simulink model "EV_model"  (R2020a)
settings: Solver=VariableStepAuto  StartTime=0  StopTime=length_DriveCycle* n_repeat  FixedStep=1  RelTol=1e-3
model workspace (MAT data in the model file):
  Af = 4
  Cd = 0.3
  DrCycles.C505 = [0 1 2 3 4 5 6 7 8 9 10 11 ... (1012 elements, 506x2)]
  DrCycles.FTP = [0 1 2 3 4 5 6 7 8 9 10 11 ... (4956 elements, 2478x2)]
  DrCycles.UDDS = [0 1 2 3 4 5 6 7 8 9 10 11 ... (2746 elements, 1373x2)]
  DrCycles.HWFET = [0 1 2 3 4 5 6 7 8 9 10 11 ... (1532 elements, 766x2)]
  DrCycles.US06 = [0 1 2 3 4 5 6 7 8 9 10 11 ... (1194 elements, 597x2)]
  DrCycles.US06City = [0 1 2 3 4 5 6 7 8 9 10 11 ... (466 elements, 233x2)]
  DrCycles.US06Hwy = [0 1 2 3 4 5 6 7 8 9 10 11 ... (742 elements, 371x2)]
  I = 1
  Kbr = 5000
  P = 20
  TimeHWFET = 765
  TimeUDDS = 1372
  TimeUS06 = 596
  axle_b = 10
  axle_k = 5000
  bevAxle_wc = 400
  bevNp = 2
  bevNs = 30
  diffRatio = 3.4
  diffRatio1 = 3.4
  motorMaxTorqueNm = [500 500 500 500 500 500 416.666666667 357.142857143 312.5 277.777777778 250 227.272727273 208.333333333 192.307692308 178.571428571 166.666666667]
  motorSpeedRadPs = [0 40 80 120 160 200 240 280 320 360 400 440 480 520 560 600]
  vehicleMass = 1500
  wheelRadius = 0.35
values from neighbouring files (symbols this model uses):
  b = 4.48/2    (= 2.24)    [NissanLeaf_input_data.m]    (also in TeslaS_input_data.m = 2.5)
  Ct = Cp_cell*rho_cell*cell_volume    (= 2759947.2)    [NissanLeaf_input_data.m]    (also in TeslaS_input_data.m = 37.7660192772)
  driving_range = 363    [NissanLeaf_input_data.m]    (also in TeslaS_input_data.m = 600)
  m = 1789    [NissanLeaf_input_data.m]    (also in TeslaS_input_data.m = 2250)
  motorMaxTorqueNm_my = [340 340 340 340 340 340 300 260  230  210 190   175 160 150 140 130 125 120]    [NissanLeaf_input_data.m]    (also in TeslaS_input_data.m = [660 660 660 660 660 660 550 475 400 325 275 225 200 175 150)
  motorSpeedRadPs_my = [1000 1500 2000 2500 3000 3250 3500 4000 4500 5000 5500 6000 6500  7000 7500 8000 8500 9000]*transRatio*2*pi/60    [NissanLeaf_input_data.m]    (also in TeslaS_input_data.m = [0 10 20 30 40 50 60 70 80 90 100 110 120 130 140 150]*0.447)
  regen_eff = 0.7    [NissanLeaf_input_data.m]    (also in TeslaS_input_data.m)
  Rt = 0.01    [NissanLeaf_input_data.m]    (also in TeslaS_input_data.m = 0.316348525327)
  T = 20    [NissanLeaf_input_data.m]    (also in TeslaS_input_data.m = 25; battery_parametrization.m)
  transRatio = 8.19    [NissanLeaf_input_data.m]    (also in TeslaS_input_data.m = 9.3)
undefined symbols (not defined in the file or in its folder): Driver, Wheels_Driver_VehDyn_Lib
libraries: autolibshared x3, simulink x2, autolibdatasheetbattery x1, autolibmappedmotor x1, autolibsharedcoupling x1, autolibshareddiff x1
(part 1 of 3)
settings Model: PauseTimes=2  Creator=ogden.michael  LastModifiedBy=marcoragone-macbookpro
settings SolverCC: AlgebraicLoopSolver=LineSearch
settings DataIOCC: ReturnWorkspaceOutputs=off
settings DebuggingCC: AlgebraicLoopMsg=none  ArithmeticOperatorsInVariantConditions=warning
settings SFSimCC: SimUseLocalCustomCode=off  CustomCodeUndefinedFunction=UseInterfaceOnly
settings RTWCC: RTWUseLocalCustomCode=off
settings CodeAppCC: StateflowObjectComments=on
settings SimscapeCC: SimscapeNormalizeSystem=off

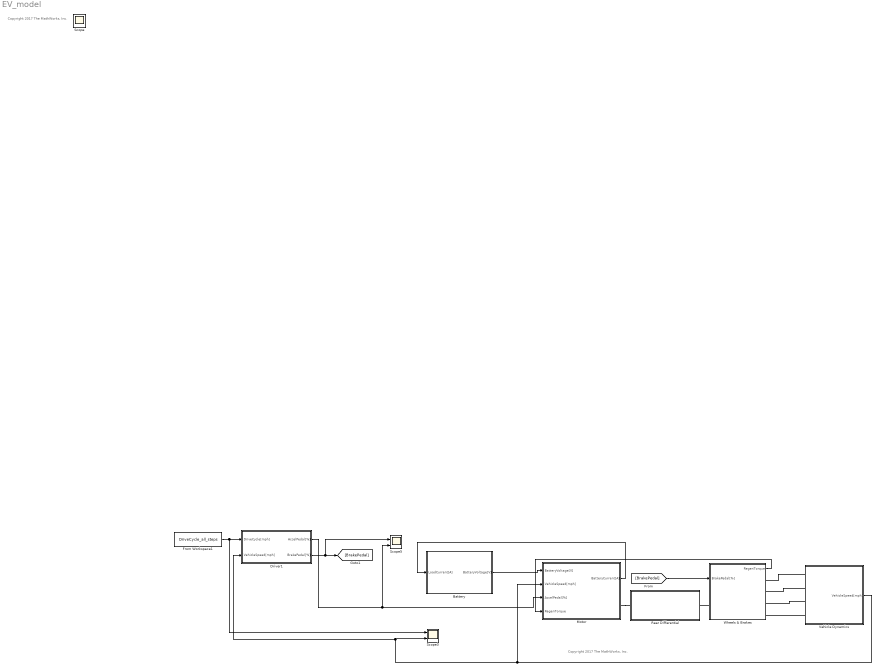
== system EV_model ==
  note: Copyright 2017 The MathWorks, Inc.
  note: Copyright 2017 The MathWorks, Inc.
  Battery : Subsystem
  Driver1 : Subsystem  AncestorBlock=Wheels_Driver_VehDyn_Lib/Driver
  From Workspace1 : FromWorkspace  VariableName=DriveCycle_all_steps
  Motor : Subsystem
  Rear Differential : Subsystem
  Scope3 : Scope  NumInputPorts=2
  Scope5 : Scope  NumInputPorts=2
  Vehicle Dynamics : Subsystem  AncestorBlock=Wheels_Driver_VehDyn_Lib/Vehicle Dynamics
  Wheels & Brakes : Subsystem  AncestorBlock=Wheels_Driver_VehDyn_Lib/Wheels & Brakes
  Scope : Scope
  wires:
  [BrakePedal] -> Wheels & Brakes/1(BrakePedal[%])
  Battery/1(BatteryVoltage[V]) -> Motor/1(BatteryVoltage[V])
  Vehicle Dynamics/1(VehicleSpeed[mph]) -> Scope3/2, Driver1/2(VehicleSpeed[mph]), Motor/2(VehicleSpeed[mph])
  Driver1/1(AccelPedal[%]) -> Scope5/2, Motor/3(AccelPedal[%])
  From Workspace1/1 -> Scope3/1, Driver1/1(" DriveCycle[mph]")
  Driver1/2(BrakePedal[%]) -> Scope5/1, [BrakePedal]
  Motor/1(BatteryCurrent[A]) -> Battery/1(LoadCurrent[A])
  Wheels & Brakes/1(RegenTorque) -> Motor/4(RegenTorque)
  connections:
  Motor/RConn1 -- Rear Differential/LConn1
  Wheels & Brakes/LConn1 -- Rear Differential/RConn1
  Vehicle Dynamics/LConn3 -- Wheels & Brakes/RConn3
  Vehicle Dynamics/LConn1 -- Wheels & Brakes/RConn1
  Vehicle Dynamics/LConn4 -- Wheels & Brakes/RConn4
  Vehicle Dynamics/LConn2 -- Wheels & Brakes/RConn2

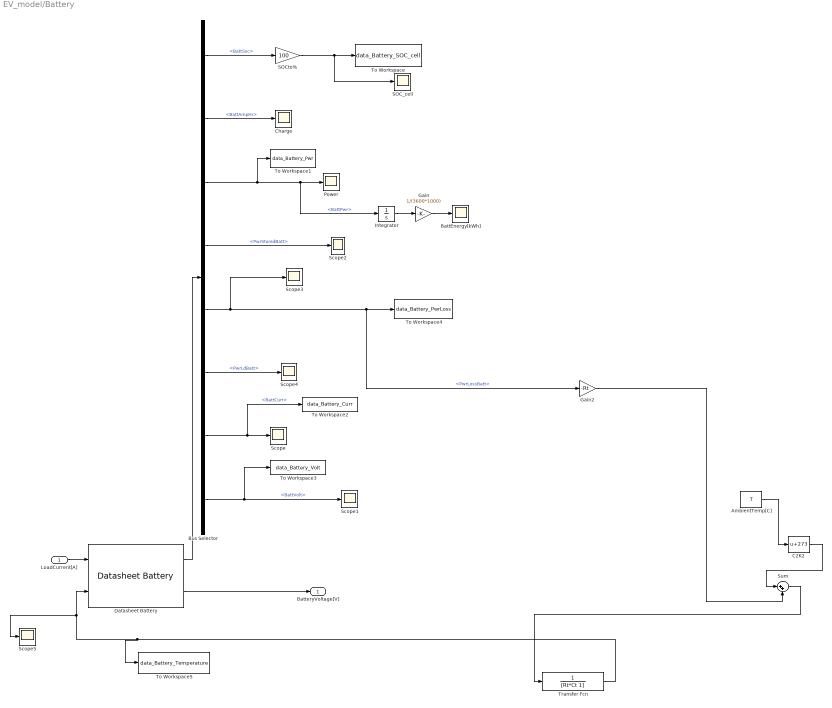
== system EV_model/Battery ==
  LoadCurrent[A] : Inport
  AmbientTemp[C] : Constant  Value=T
  BattEnergy[kWh] : Scope
  Bus Selector : BusSelector  OutputSignals=BattSoc,BattAmpHr,BattPwr,PwrInfo.PwrStored.PwrStoredBatt,PwrInfo.PwrNotTrnsfrd.PwrLossBatt,PwrInfo.PwrTrnsfrd.PwrLdBatt,BattCurr,BattVolt
  C2K2 : Bias  Bias=273
  Charge : Scope
  Datasheet Battery : autolibdatasheetbattery/Datasheet Battery  CapacityCtrl=Parameter  OutputVlt=Unfiltered  BattChargeMax=BattChargeMax  Em=Em  CapLUTBp=CapLUTBp  RInt=RInt  BattTempBp=BattTempBp  CapSOCBp=CapSOCBp  Ns=Ns  Np=Np  BattCapInit=BattCapInit  Tc=1/1000  Vinit=4.221  RefBlkName='autolibdatasheetbattery/Datasheet Battery'
      settings: SourceProductBaseCode=PW
  Gain : Gain  Gain=1/(3600*1000)
  Gain2 : Gain  Gain=-Rt
  Integrator : Integrator
  Power : Scope
  SOC_cell : Scope
  SOCto% : Gain  Gain=100
  Scope{,1..5} (6 alike) : Scope
  Sum : Sum  Inputs=|++
  To Workspace : ToWorkspace  VariableName=data_Battery_SOC_cell  SaveFormat=Timeseries  SampleTime=-1
  To Workspace1 : ToWorkspace  VariableName=data_Battery_Pwr  SaveFormat=Timeseries  SampleTime=-1
  To Workspace2 : ToWorkspace  VariableName=data_Battery_Curr  SaveFormat=Timeseries  SampleTime=-1
  To Workspace3 : ToWorkspace  VariableName=data_Battery_Volt  SaveFormat=Timeseries  SampleTime=-1
  To Workspace4 : ToWorkspace  VariableName=data_Battery_PwrLoss  SaveFormat=Timeseries  SampleTime=-1
  To Workspace5 : ToWorkspace  VariableName=data_Battery_Temperature  SaveFormat=Timeseries  SampleTime=-1
  Transfer Fcn : TransferFcn  Numerator=[0 1]  Denominator=[Rt*Ct 1]
  BatteryVoltage[V] : Outport  VectorParamsAs1DForOutWhenUnconnected=off
  wires:
  Datasheet Battery/1 -> Bus Selector/1
  Datasheet Battery/2 -> BatteryVoltage[V]/1
  SOCto%/1 -> SOC_cell/1, To Workspace/1
  Bus Selector/1 -> SOCto%/1  "<BattSoc>"
  LoadCurrent[A]/1 -> Datasheet Battery/1
  Bus Selector/2 -> Charge/1  "<BattAmpHr>"
  Bus Selector/3 -> Integrator/1, Power/1, To Workspace1/1  "<BattPwr>"
  Bus Selector/7 -> Scope/1, To Workspace2/1  "<BattCurr>"
  Bus Selector/8 -> Scope1/1, To Workspace3/1  "<BattVolt>"
  Bus Selector/4 -> Scope2/1  "<PwrStoredBatt>"
  Bus Selector/6 -> Scope4/1  "<PwrLdBatt>"
  Integrator/1 -> Gain/1
  Gain/1 -> BattEnergy[kWh]/1
  Gain2/1 -> Sum/2
  C2K2/1 -> Sum/1
  AmbientTemp[C]/1 -> C2K2/1
  Bus Selector/5 -> Scope3/1, Gain2/1, To Workspace4/1  "<PwrLossBatt>"
  Sum/1 -> Transfer Fcn/1
  Transfer Fcn/1 -> To Workspace5/1, Datasheet Battery/2, Scope5/1

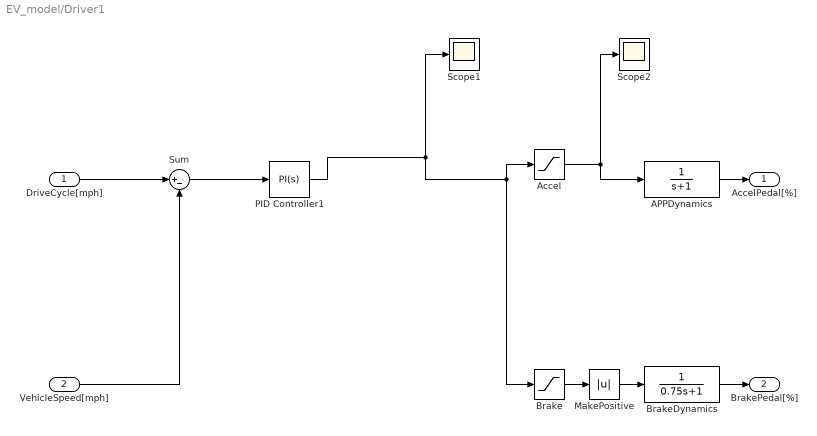
== system EV_model/Driver1 ==
  " DriveCycle[mph]" : Inport
  VehicleSpeed[mph] : Inport  Port=2
  APPDynamics : TransferFcn  Denominator=[1 1]
  Accel : Saturate  UpperLimit=100  LowerLimit=0
  Brake : Saturate  UpperLimit=0  LowerLimit=-100
  BrakeDynamics : TransferFcn  Denominator=[0.75 1]
  MakePositive : Abs
  PID Controller1 : simulink/Continuous/PID Controller  Controller=PI  Form=Parallel  TimeDomain=Continuous-time  UseExternalTs=off  SampleTime=-1  IntegratorMethod=Forward Euler  FilterMethod=Forward Euler  ControllerParametersSource=internal  P=20  I=1  D=0.1  UseFilter=on  N=100  TunerSelectOption=Frequency Response Based  InitialConditionSource=internal  InitialConditionForIntegrator=0  InitialConditionForFilter=0  DifferentiatorICPrevScaledInput=0  ExternalReset=none  TrackingMode=off  Kt=1  LimitOutput=off  UpperSaturationLimit=inf  LowerSaturationLimit=-inf  LinearizeAsGain=on  AntiWindupMode=none  Kb=1  POutMin=[]  POutMax=[]  IOutMin=[]  IOutMax=[]  DOutMin=[]  DOutMax=[]  NOutMin=[]  NOutMax=[]  SumOutMin=[]  SumOutMax=[]  SaturationOutMin=[]  SaturationOutMax=[]  PParamMin=[]  PParamMax=[]  IParamMin=[]  IParamMax=[]  DParamMin=[]  DParamMax=[]  NParamMin=[]  NParamMax=[]  KbParamMin=[]  KbParamMax=[]  KtParamMin=[]  KtParamMax=[]  KbOutMin=[]  KbOutMax=[]  KtOutMin=[]  KtOutMax=[]  IntegratorOutMin=[]  IntegratorOutMax=[]  FilterOutMin=[]  FilterOutMax=[]  SumI1OutMin=[]  SumI1OutMax=[]  SumI2OutMin=[]  SumI2OutMax=[]  SumI3OutMin=[]  SumI3OutMax=[]  SumI4OutMin=[]  SumI4OutMax=[]  SumDOutMin=[]  SumDOutMax=[]  DifferentiatorOutMin=[]  DifferentiatorOutMax=[]  FilterDiffOutCoefMin=[]  FilterDiffOutCoefMax=[]  ReciprocalOutMin=[]  ReciprocalOutMax=[]  SumDenOutMin=[]  SumDenOutMax=[]  SumNumOutMin=[]  SumNumOutMax=[]  DivideOutMin=[]  DivideOutMax=[]  UdiffTsProdOutMin=[]  UdiffTsProdOutMax=[]  NTsProdOutMin=[]  NTsProdOutMax=[]  UintegralTsProdOutMin=[]  UintegralTsProdOutMax=[]  UngainTsProdOutMin=[]  UngainTsProdOutMax=[]  IntegratorContinuousStateAttributes=''  IntegratorStateMustResolveToSignalObject=off  IntegratorRTWStateStorageClass=Auto  FilterContinuousStateAttributes=''  FilterStateMustResolveToSignalObject=off  FilterRTWStateStorageClass=Auto  ParallelPVariant=InternalParameters  IdealPVariant=Disabled  IVariant=InternalParameters  DVariant=Disabled  IntegratorVariant=Continuous  SatVariant=Disabled  AWVariant=Passthrough  PCopyVariant=Disabled  TRVariant=Disabled  FdbkBlocksVariant=Forward  IdealPFdbkVariant=Disabled  SatFdbkVariant=Disabled  DerivativeFilterVariant=Disabled  NVariant=Disabled  NCopyVariant=Disabled_SignalSpec  FilterICVariant=Disabled  IntegratorICVariant=InternalICs  ExternalResetVariant=Disabled  TRSumVariant=Passthrough  SumFdbkVariant=Disabled  SumVariant=Sum_PI  TsampFilterVariant=InternalTs  TsampNgainVariant=Passthrough  TsampIntegralVariant=Passthrough
  Scope1 : Scope
  Scope2 : Scope
  Sum : Sum  Inputs=|+-
  AccelPedal[%] : Outport  VectorParamsAs1DForOutWhenUnconnected=off
  BrakePedal[%] : Outport  Port=2  VectorParamsAs1DForOutWhenUnconnected=off
  wires:
  MakePositive/1 -> BrakeDynamics/1
  " DriveCycle[mph]"/1 -> Sum/1
  VehicleSpeed[mph]/1 -> Sum/2
  Brake/1 -> MakePositive/1
  Accel/1 -> Scope2/1, APPDynamics/1
  APPDynamics/1 -> AccelPedal[%]/1
  PID Controller1/1 -> Accel/1, Brake/1, Scope1/1
  Sum/1 -> PID Controller1/1
  BrakeDynamics/1 -> BrakePedal[%]/1

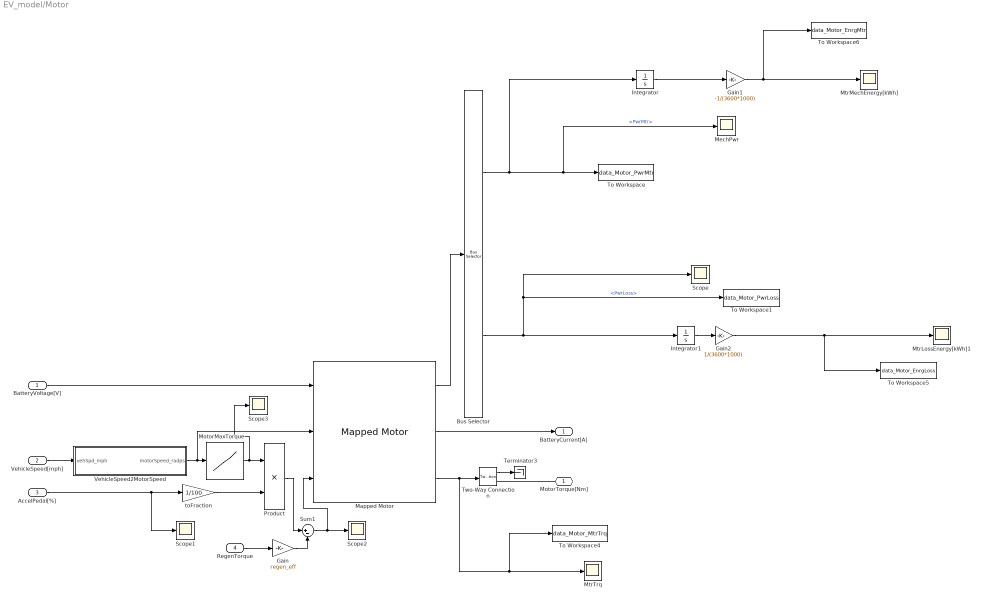
== system EV_model/Motor ==
  BatteryVoltage[V] : Inport
  VehicleSpeed[mph] : Inport  Port=2
  AccelPedal[%] : Inport  Port=3
  RegenTorque : Inport  Port=4
  Bus Selector : BusSelector  OutputSignals=PwrInfo.PwrTrnsfrd.PwrMtr,PwrInfo.PwrNotTrnsfrd.PwrLoss
  Gain : Gain  Gain=regen_eff
  Gain1 : Gain  Gain=-1/(3600*1000)
  Gain2 : Gain  Gain=1/(3600*1000)
  Integrator : Integrator
  Integrator1 : Integrator
  Mapped Motor : autolibmappedmotor/Mapped Motor  port_config=Speed  param_by=Tabulated torque-speed envelope  w_t=motorSpeedRadPs_my  T_t=motorMaxTorqueNm_my  torque_max=torque_max  power_max=power_max  Tc=0.02  param_loss=Single efficiency measurement  eff=100  w_eff=375  T_eff=0.08  Piron=0  Pbase=0  w_eff_bp=[-8000 -4000 0 4000 8000]  T_eff_bp=[0 0.03 0.06 0.09]  Temp_eff_bp=[233.15 293.15 373.15]  losses_table=[1.49 1.67 2.21 3.10; 0.42 0.69 1.14 2.03; 0.06 0.24 0.78 1.68; 0.42 0.69 1.14 2.03; 1.49 1.67 2.21 3.10]  losses_table_3d=cat(3,1.05*[1.49 1.67 2.21 3.10; 0.42 0.69 1.14 2.03; 0.06 0.24 0.78 1.68; 0.42 0.69 1.14 2.03; 1.49 1.67 2.21 3.10],[1.49 1.67 2.21 3.10; 0.42 0.69 1.14 2.03; 0.06 0.24 0.78 1.68; 0.42 0.69 1.14 2.03; 1.49 1.67 2.21 3.10],1.03*[1.49 1.67 2.21 3.10; 0.42 0.69 1.14 2.03; 0.06 0.24 0.78 1.68; 0.42 0.69 1.14 2.03; 1.49 1.67 2.21 3.10])  efficiency_table=[95 95 95 95; 95 95 95 95; 95 95 95 95; 95 95 95 95; 95 95 95 95]  efficiency_table_3d=cat(3,90*ones(5,4),95*ones(5,4),92*ones(5,4))  J=5e-6  b=1e-5  omega_o=0  T_t_extended=[125 150 175 200 225 275 325 400 475 550 660 660 660 660 660 660 660 660 660 660 660 550 475 400 325 275 225 200 175 150 125]  w_t_extended=[-2711.15217391304 -2530.40869565217 -2349.6652173913 -2168.92173913043 -1988.17826086957 -1807.4347826087 -1626.69130434783 -1445.94782608696 -1265.20434782609 -1084.46086956522 -903.717391304348 -722.973913043478 -542.230434782609 -361.486956521739 -180.74347826087 0 180.74347826087 361.486956521739 542.230434782609 722.973913043478 903.717391304348 1084.46086956522 1265.20434782609 1445.94782608696 1626.69130434783 1807.4347826087 1988.17826086957 2168.92173913043 2349.6652173913 2530.40869565217 2711.15217391304]  KLossIron=0  KLossCopper=0  x_w_eff_vec=[-8000 -4000 0 4000 8000]  x_T_eff_vec=[-0.09 -0.06 -0.03 0 0.03 0.06 0.09]  x_tmp_eff_vec=[233.15 293.15 373.15]  x_losses_mat=[3.1 2.21 1.67 1.49 1.67 2.21 3.1;2.03 1.14 0.69 0.42 0.69 1.14 2.03;1.68 0.78 0.24 0.06 0.24 0.78 1.68;2.03 1.14 0.69 0.42 0.69 1.14 2.03;3.1 2.21 1.67 1.49 1.67 2.21 3.1]  x_losses_mat_3d=cat(3,[3.255 2.3205 1.7535 1.5645 1.7535 2.3205 3.255;2.1315 1.197 0.7245 0.441 0.7245 1.197 2.1315;1.764 0.819 0.252 0.063 0.252 0.819 1.764;2.1315 1.197 0.7245 0.441 0.7245 1.197 2.1315;3.255 2.3205 1.7535 1.5645 1.7535 2.3205 3.255],[3.1 2.21 1.67 1.49 1.67 2.21 3.1;2.03 1.14 0.69 0.42 0.69 1.14 2.03;1.68 0.78 0.24 0.06 0.24 0.78 1.68;2.03 1.14 0.69 0.42 0.69 1.14 2.03;3.1 2.21 1.67 1.49 1.67 2.21 3.1],[3.193 2.2763 1.7201 1.5347 1.7201 2.2763 3.193;2.0909 1.1742 0.7107 0.4326 0.7107 1.1742 2.0909;1.7304 0.8034 0.2472 0.0618 0.2472 0.8034 1.7304;2.0909 1.1742 0.7107 0.4326 0.7107 1.1742 2.0909;3.193 2.2763 1.7201 1.5347 1.7201 2.2763 3.193])  CalLossMapData={}  CalLossWithTempMapData={}  aMode=aMode  RefBlkName='autolibmappedmotor/Mapped Motor'
      settings: SourceProductBaseCode=PW,MT,VE,VP
  MechPwr : Scope
  MotorMaxTorque : Lookup_n-D  NumberOfTableDimensions=1  BreakpointsForDimension1=motorSpeedRadPs_my  Table=motorMaxTorqueNm_my  ExtrapMethod=Clip  InternalRulePriority=Speed  RndMeth=Simplest  InputSameDT=on
  MtrLossEnergy[kWh]1 : Scope
  MtrMechEnergy[kWh] : Scope
  MtrTrq : Scope
  Product : Product
  Scope{,1..3} (4 alike) : Scope
  Sum1 : Sum  Inputs=|+-
  Terminator3 : Terminator
  To Workspace : ToWorkspace  VariableName=data_Motor_PwrMtr  SaveFormat=Timeseries  SampleTime=-1
  To Workspace1 : ToWorkspace  VariableName=data_Motor_PwrLoss  SaveFormat=Timeseries  SampleTime=-1
  To Workspace4 : ToWorkspace  VariableName=data_Motor_MtrTrq  SaveFormat=Timeseries  SampleTime=-1
  To Workspace5 : ToWorkspace  VariableName=data_Motor_EnrgLoss  SaveFormat=Timeseries  SampleTime=-1
  To Workspace6 : ToWorkspace  VariableName=data_Motor_EnrgMtr  SaveFormat=Timeseries  SampleTime=-1
  Two-Way Connectio n : TwoWayConnection
  VehicleSpeed2MotorSpeed : Subsystem
  toFraction : Gain  Gain=1/100
  MotorTorque[Nm] : PMIOPort  Side=Right
  BatteryCurrent[A] : Outport  VectorParamsAs1DForOutWhenUnconnected=off
  wires:
  BatteryVoltage[V]/1 -> Mapped Motor/1
  Mapped Motor/2 -> BatteryCurrent[A]/1
  VehicleSpeed[mph]/1 -> VehicleSpeed2MotorSpeed/1(vehSpd_mph)
  VehicleSpeed2MotorSpeed/1(motorSpeed_radps) -> Mapped Motor/2, MotorMaxTorque/1
  Mapped Motor/1 -> Bus Selector/1
  Two-Way Connectio n/1 -> Terminator3/1
  MotorMaxTorque/1 -> Scope3/1, Product/1
  AccelPedal[%]/1 -> Scope1/1, toFraction/1
  toFraction/1 -> Product/2
  Bus Selector/1 -> Integrator/1, MechPwr/1, To Workspace/1  "<PwrMtr>"
  Mapped Motor/3 -> MtrTrq/1, To Workspace4/1, Two-Way Connectio n/1
  Product/1 -> Sum1/1
  Sum1/1 -> Mapped Motor/3, Scope2/1
  Gain/1 -> Sum1/2
  RegenTorque/1 -> Gain/1
  Gain1/1 -> To Workspace6/1, MtrMechEnergy[kWh]/1
  Integrator/1 -> Gain1/1
  Integrator1/1 -> Gain2/1
  Bus Selector/2 -> Scope/1, To Workspace1/1, Integrator1/1  "<PwrLoss>"
  Gain2/1 -> MtrLossEnergy[kWh]1/1, To Workspace5/1
  connections:
  MotorTorque[Nm]/RConn1 -- Two-Way Connectio n/RConn1

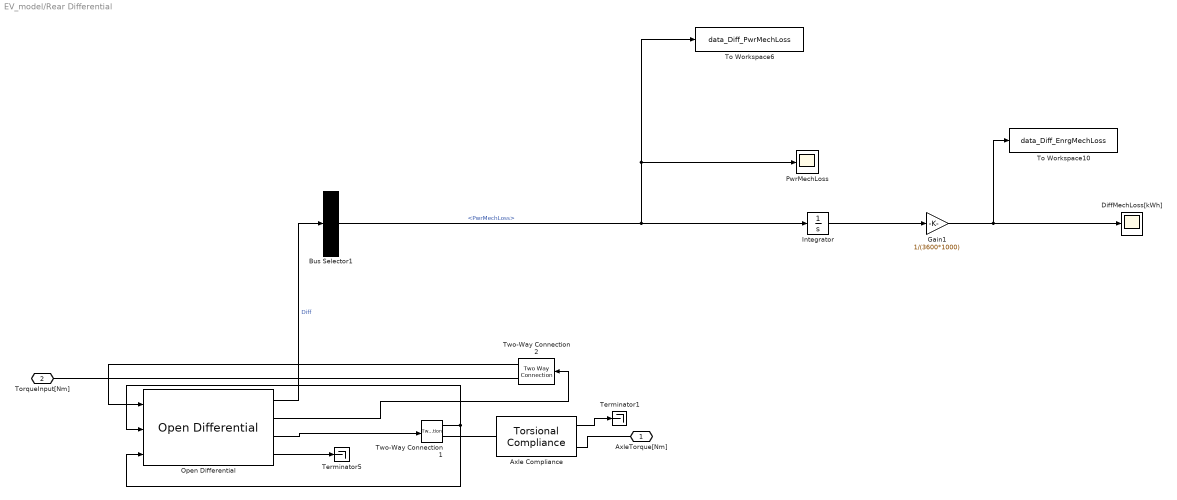
== system EV_model/Rear Differential ==
  Axle Compliance : autolibsharedcoupling/Torsional Compliance  port_config=Two-way connection  extInfo=on  k=axle_k  b=axle_b  theta_o=0  domega_o=0  omega_c=bevAxle_wc  blkID=0  aMode=1
      settings: SourceProductBaseCode=PW,MT,VE,VP
  Bus Selector1 : BusSelector  OutputSignals=PwrInfo.PwrNotTrnsfrd.PwrMechLoss
  DiffMechLoss[kWh] : Scope
  Gain1 : Gain  Gain=1/(3600*1000)
  Integrator : Integrator
  Open Differential : autolibshareddiff/Open Differential  DiffEffModelPopup=Constant  InterpMethod=Linear point-slope  extTamb=off  shaftSwitchMask=To the left of center-line  Ndiff=transRatio  Jd=.025  bd=1e-3  Jw1=.01  bw1=1e-3  Jw2=.01  bw2=1e-3  omegaw1o=0  omegaw2o=0  eta=transEff  eta_tbl=reshape([0.64 0.76 0.8 0.81 0.83 0.84 0.84 0.56 0.73 0.78 0.8 0.83 0.84 0.84 0.54 0.71 0.77 0.8 0.82 0.84 0.84 0.53 0.71 0.77 0.8 0.83 0.84 0.84 0.51 0.71 0.77 0.8 0.83 0.84 0.85 0.52 0.7 0.77 0.8 0.83 0.84 0.85 0.51 0.71 0.76 0.79 0.83 0.84 0.85 0.5 0.69 0.76 0.79 0.82 0.84 0.85 0.45 0.68 0.75 0.78 0.82 0.84 0.85 0.43 0.67 0.74 0.78 0.81 0.83 0.84 0.38 0.63 0.71 0.75 0.8 0.82 0.83 0.81 0.86 0.88 0.89 0.89 0.89 0.9 0.77 0.85 0.87 0.88 0.89 0.9 0.9 0.72 0.82 0.86 0.87 0.88 0.89 0.9 0.68 0.8 0.84 0.86 0.88 0.89 0.89 0.67 0.8 0.84 0.86 0.88 0.89 0.9 0.67 0.8 0.84 0.86 0.88 0.89 0.9 0.65 0.8 0.84 0.86 0.88 0.89 0.9 0.64 0.79 0.83 0.86 0.88 0.89 0.9 0.63 0.78 0.83 0.86 0.88 0.89 0.9 0.59 0.76 0.82 0.85 0.87 0.89 0.9 0.53 0.73 0.8 0.83 0.86 0.88 0.89], 7, 11, 2)  Trq_bpts=[25, 50, 75, 100, 150, 200, 250]  omega_bpts=[52.4 78.5 105 131 157 183 209 262 314 419 524]  Temp_bpts=[290 358]  Tamb=T+273  maxAbsSpd=5e3  aMode=aMode
      settings: SourceProductBaseCode=PW,MT,VE,VP
  PwrMechLoss : Scope
  Terminator1 : Terminator
  Terminator5 : Terminator
  To Workspace10 : ToWorkspace  VariableName=data_Diff_EnrgMechLoss  SaveFormat=Timeseries  SampleTime=-1
  To Workspace6 : ToWorkspace  VariableName=data_Diff_PwrMechLoss  SaveFormat=Timeseries  SampleTime=-1
  Two-Way Connection1 : TwoWayConnection
  Two-Way Connection2 : TwoWayConnection
  AxleTorque[Nm] : PMIOPort  Side=Right
  TorqueInput[Nm] : PMIOPort  Port=2  Side=Left
  wires:
  Open Differential/3 -> Two-Way Connection1/1
  Open Differential/4 -> Terminator5/1
  Open Differential/2 -> Two-Way Connection2/1
  Two-Way Connection2/1 -> Open Differential/1
  Two-Way Connection1/1 -> Open Differential/2, Open Differential/3
  Open Differential/1 -> Bus Selector1/1  "Diff"
  Integrator/1 -> Gain1/1
  Gain1/1 -> To Workspace10/1, DiffMechLoss[kWh]/1
  Bus Selector1/1 -> To Workspace6/1, PwrMechLoss/1, Integrator/1  "<PwrMechLoss>"
  Axle Compliance/1 -> Terminator1/1
  connections:
  Axle Compliance/LConn1 -- Two-Way Connection1/RConn1
  TorqueInput[Nm]/RConn1 -- Two-Way Connection2/RConn1
  AxleTorque[Nm]/RConn1 -- Axle Compliance/RConn1

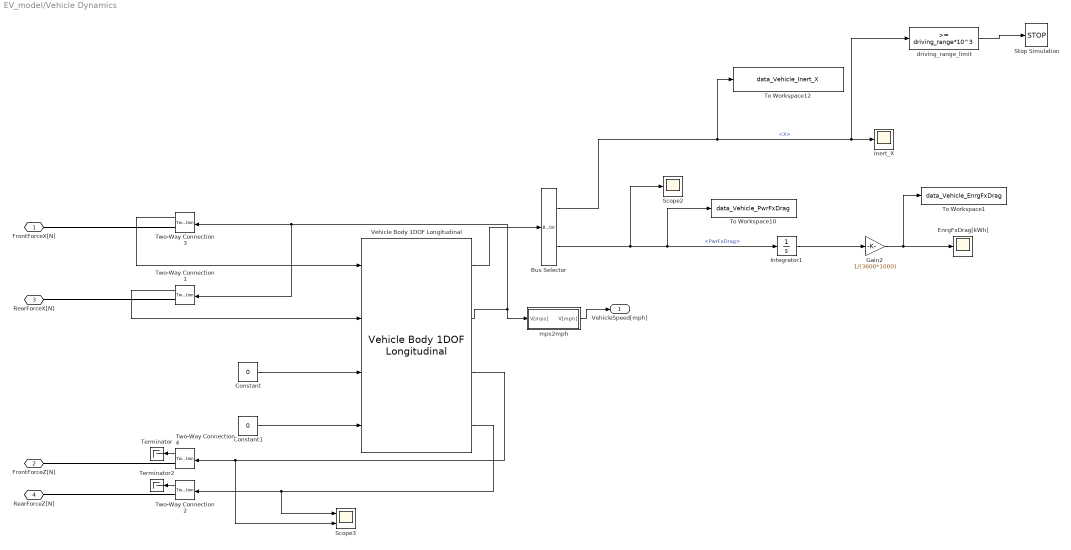
== system EV_model/Vehicle Dynamics ==
  Bus Selector : BusSelector  OutputSignals=InertFrm.Cg.Disp.X,PwrInfo.PwrNotTrnsfrd.PwrFxDrag
  Constant : Constant  Value=0
  Constant1 : Constant  Value=0
  EnrgFxDrag[kWh] : Scope
  Gain2 : Gain  Gain=1/(3600*1000)
  Inert_X : Scope
  Integrator1 : Integrator
  Scope2 : Scope
  Scope3 : Scope  NumInputPorts=2
  Stop Simulation : Stop
  Terminator : Terminator
  Terminator2 : Terminator
  To Workspace1 : ToWorkspace  VariableName=data_Vehicle_EnrgFxDrag  SaveFormat=Timeseries  SampleTime=-1
  To Workspace10 : ToWorkspace  VariableName=data_Vehicle_PwrFxDrag  SaveFormat=Timeseries  SampleTime=-1
  To Workspace12 : ToWorkspace  VariableName=data_Vehicle_Inert_X  SaveFormat=Timeseries  SampleTime=-1
  Two-Way Connection{1..4} (4 alike) : TwoWayConnection
  Vehicle Body 1DOF Longitudinal : autolibshared/Vehicle Body 1DOF Longitudinal  VariantControl=SL  extFMode=off  extMMode=off  extTamb=off  wind3D=off  aMode=aMode  NF=2  NR=2  m=m  a=a  b=b  h=h  Cd=Cdrag  Cl=0  Cpm=0  Af=Af  x_o=0  xdot_o=0  Pabs=101325  T=T+273  g=9.81
      settings: SourceProductBaseCode=PW,MT,VE,VP
  driving_range_limit : simulink/Logic and Bit Operations/Compare To Constant  relop=>=  const=driving_range*10^3  OutDataTypeStr=boolean
  mps2mph : Subsystem
  FrontForceX[N] : PMIOPort  Side=Left
  FrontForceZ[N] : PMIOPort  Port=2  Side=Left
  RearForceX[N] : PMIOPort  Port=3  Side=Left
  RearForceZ[N] : PMIOPort  Port=4  Side=Left
  VehicleSpeed[mph] : Outport  VectorParamsAs1DForOutWhenUnconnected=off
  wires:
  Constant1/1 -> Vehicle Body 1DOF Longitudinal/4
  Vehicle Body 1DOF Longitudinal/2 -> Two-Way Connection1/1, Two-Way Connection3/1, mps2mph/1(V[mps])
  Vehicle Body 1DOF Longitudinal/1 -> Bus Selector/1
  Vehicle Body 1DOF Longitudinal/3 -> Scope3/2, Two-Way Connection4/1
  Vehicle Body 1DOF Longitudinal/4 -> Scope3/1, Two-Way Connection2/1
  Two-Way Connection3/1 -> Vehicle Body 1DOF Longitudinal/1
  Two-Way Connection1/1 -> Vehicle Body 1DOF Longitudinal/2
  Two-Way Connection4/1 -> Terminator/1
  Two-Way Connection2/1 -> Terminator2/1
  mps2mph/1(V[mph]) -> VehicleSpeed[mph]/1
  Constant/1 -> Vehicle Body 1DOF Longitudinal/3
  Bus Selector/1 -> To Workspace12/1, driving_range_limit/1, Inert_X/1  "<X>"
  Gain2/1 -> To Workspace1/1, EnrgFxDrag[kWh]/1
  Integrator1/1 -> Gain2/1
  Bus Selector/2 -> Scope2/1, To Workspace10/1, Integrator1/1  "<PwrFxDrag>"
  driving_range_limit/1 -> Stop Simulation/1
  connections:
  FrontForceX[N]/RConn1 -- Two-Way Connection3/RConn1
  FrontForceZ[N]/RConn1 -- Two-Way Connection4/RConn1
  RearForceX[N]/RConn1 -- Two-Way Connection1/RConn1
  RearForceZ[N]/RConn1 -- Two-Way Connection2/RConn1
